simulink model "DomsProject_change_from_deg_to_rad"  (Simulink 8.7)
settings: Solver=VariableStepAuto  StartTime=0.0  StopTime=20  RelTol=1e-3
model workspace (MATLAB code in the model file):
  | J=0.000027; % Inertia kg/m^2
  | R=9.02; % Resistance Ohms
  | b=0.07; % Viscus damping NM/(rads/s)
  | Kt=0.63; % Torque Constant Nm/A
  | Ke=0.39; % Voltage constant V/(Rads/s)
  | L=0.0187; % Inductance H
  | m=0.1; % mass KG
  | G1= 0.1 % Saturation gain for friction model
  | g=9.81 % gravity m/sec^2
  | l=0.15 % length of arm in metres
libraries: simulink x2
settings Model: Creator=Lara  LastModifiedBy=mmdclm
settings DataIOCC: LimitDataPoints=off  SaveFormat=Dataset
settings DebuggingCC: UnderspecifiedInitializationDetection=Simplified  MergeDetectMultiDrivingBlocksExec=error
settings HardwareCC: ProdBitPerPointer=64  ProdLargestAtomicFloat=Float  ProdIntDivRoundTo=Zero  ProdEndianess=LittleEndian  ProdWordSize=64  ProdHWDeviceType=Intel->x86-64 (Windows64)
settings ModelReferenceCC: PropagateSignalLabelsOutOfModel=on
settings ConfigComp: CovModelRefEnable=off

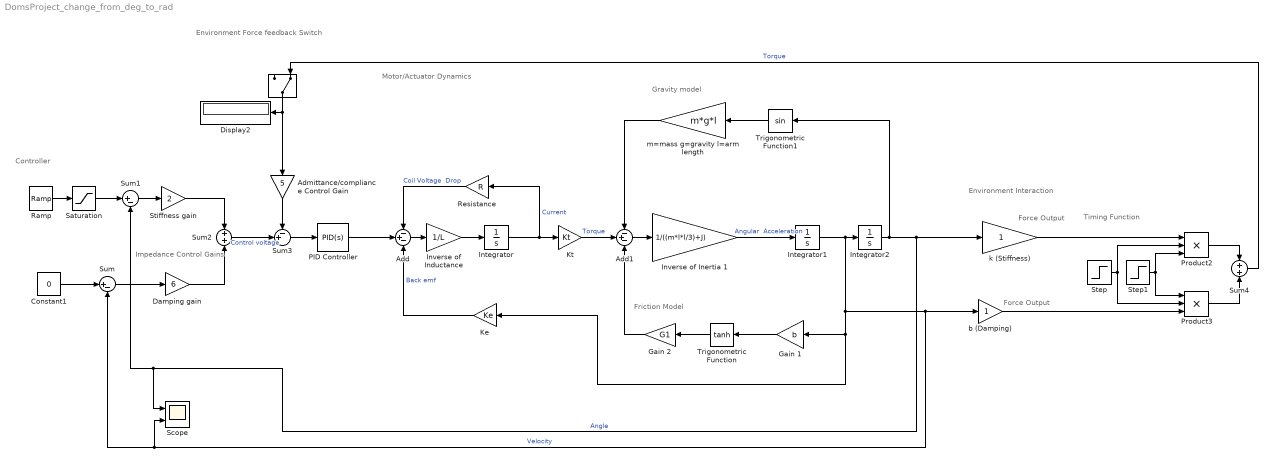
== system DomsProject_change_from_deg_to_rad ==
  note: Impedance Control
      | Gains
  note: Timing Function
  note: Force Output
  note: Force Output
  note: Environment
      | Force feedback
      | Switch
  note: Environment Interaction
  note: Motor/Actuator Dynamics
  note: Controller
  note: Gravity model
  note: Friction Model
  " " : ManualSwitch  CurrentSetting=0
  Add : Sum  Inputs=-+-
  Add1 : Sum  Inputs=-+-
  Admittance/compliance Control Gain : Gain  Gain=5
  Constant1 : Constant  Value=0
  Damping gain : Gain  Gain=6
  Display2 : Display
  Gain 1 : Gain  Gain=b
  Gain 2 : Gain  Gain=G1
  Integrator : Integrator
  Integrator1 : Integrator
  Integrator2 : Integrator
  Inverse of Inductance : Gain  Gain=1/L
  Inverse of Inertia 1 : Gain  Gain=1/((m*l*l/3)+J)
  "Ke " : Gain  Gain=Ke
  "Kt " : Gain  Gain=Kt
  PID Controller : simulink/Continuous/PID Controller  Controller=PID  TimeDomain=Continuous-time  SampleTime=-1  IntegratorMethod=Forward Euler  FilterMethod=Forward Euler  Form=Parallel  UseFilter=on  ControllerParametersSource=internal  P=0  I=0.731381886063385  D=0  N=100  InitialConditionSource=internal  InitialConditionForIntegrator=0  InitialConditionForFilter=0  ExternalReset=none  LimitOutput=off  UpperSaturationLimit=inf  LowerSaturationLimit=-inf  LinearizeAsGain=on  AntiWindupMode=none  Kb=1  TrackingMode=off  Kt=1  PParamMin=[]  PParamMax=[]  IParamMin=[]  IParamMax=[]  DParamMin=[]  DParamMax=[]  NParamMin=[]  NParamMax=[]  KbParamMin=[]  KbParamMax=[]  KtParamMin=[]  KtParamMax=[]  POutMin=[]  POutMax=[]  IOutMin=[]  IOutMax=[]  DOutMin=[]  DOutMax=[]  NOutMin=[]  NOutMax=[]  KbOutMin=[]  KbOutMax=[]  KtOutMin=[]  KtOutMax=[]  IntegratorOutMin=[]  IntegratorOutMax=[]  FilterOutMin=[]  FilterOutMax=[]  SumOutMin=[]  SumOutMax=[]  SumI1OutMin=[]  SumI1OutMax=[]  SumI2OutMin=[]  SumI2OutMax=[]  SumI3OutMin=[]  SumI3OutMax=[]  SumDOutMin=[]  SumDOutMax=[]  SaturationOutMin=[]  SaturationOutMax=[]  IntegratorContinuousStateAttributes=''  IntegratorStateMustResolveToSignalObject=off  IntegratorRTWStateStorageClass=Auto  FilterContinuousStateAttributes=''  FilterStateMustResolveToSignalObject=off  FilterRTWStateStorageClass=Auto  DifferentiatorICPrevScaledInput=0  DifferentiatorOutMin=[]  DifferentiatorOutMax=[]
  Product2 : Product  Inputs=3
  Product3 : Product  Inputs=3
  Ramp : simulink/Sources/Ramp  slope=10  start=0  X0=0
  "Resistance " : Gain  Gain=R
  Saturation : Saturate  UpperLimit=3.142
  Scope : Scope  NumInputPorts=2
  Step : Step  SampleTime=0
  Step1 : Step  Time=2  Before=1  After=0  SampleTime=0
  Stiffness gain : Gain  Gain=2
  Sum : Sum  Inputs=|+-
  Sum1 : Sum  Inputs=|+-
  Sum2 : Sum  Inputs=+|+
  Sum3 : Sum  Inputs=-+|
  Sum4 : Sum  Inputs=+|+
  Trigonometric Function : Trigonometry  Operator=tanh
  Trigonometric Function1 : Trigonometry
  b (Damping) : Gain
  k (Stiffness) : Gain
  m=mass g=gravity l=arm length : Gain  Gain=m*g*l
  wires:
  Constant1/1 -> Sum/1
  Sum/1 -> Damping gain/1
  Sum1/1 -> Stiffness gain/1
  Stiffness gain/1 -> Sum2/1
  Damping gain/1 -> Sum2/2
  Add1/1 -> Inverse of Inertia 1/1
  Trigonometric Function1/1 -> m=mass g=gravity l=arm length/1
  "Kt "/1 -> Add1/2  "Torque"
  "Ke "/1 -> Add/3  "Back emf"
  Integrator/1 -> "Resistance "/1, "Kt "/1  "Current"
  Integrator1/1 -> Scope/2, Sum/2, b (Damping)/1, "Ke "/1, Gain 1/1, Integrator2/1  "Velocity"
  "Resistance "/1 -> Add/1  "Coil Voltage  Drop"
  Inverse of Inertia 1/1 -> Integrator1/1  "Angular  Acceleration"
  Add/1 -> Inverse of Inductance/1
  Inverse of Inductance/1 -> Integrator/1
  Integrator2/1 -> k (Stiffness)/1, Scope/1, Sum1/2, Trigonometric Function1/1  "Angle"
  Sum2/1 -> Sum3/2  "Control voltage"
  Gain 1/1 -> Trigonometric Function/1
  Trigonometric Function/1 -> Gain 2/1
  Sum3/1 -> PID Controller/1
  PID Controller/1 -> Add/2
  Ramp/1 -> Saturation/1
  " "/1 -> Display2/1, Admittance/compliance Control Gain/1
  Step1/1 -> Product3/1, Product2/3
  Step/1 -> Product3/2, Product2/2
  m=mass g=gravity l=arm length/1 -> Add1/1
  Saturation/1 -> Sum1/1
  Sum4/1 -> " "/2  "Torque"
  Admittance/compliance Control Gain/1 -> Sum3/1
  Gain 2/1 -> Add1/3
  k (Stiffness)/1 -> Product2/1
  b (Damping)/1 -> Product3/3
  Product3/1 -> Sum4/2
  Product2/1 -> Sum4/1
